simulink model "xxxx"  (R2025a)
settings: Solver=ode23t  StartTime=0.0  StopTime=10.0  RelTol=1e-3  AbsTol=1e-3  EnableMultiTasking=on
values from neighbouring files (symbols this model uses):
  FemurHeight = 0.25    [xxxx_ini.m]
  FemurRadius = 0.05    [xxxx_ini.m]
  FootDepth = 0.25    [xxxx_ini.m]
  FootHeight = 0.05    [xxxx_ini.m]
  FootWidth = 0.1    [xxxx_ini.m]
  PelvisHorizontalPositionInit = FemurHeight * sin(HipRadInit)                               + TibiaHeight * sin(HipRadInit + KneeRadInit)    [xxxx_ini.m]
  PelvisRadius = 0.15    [xxxx_ini.m]
  PelvisVerticalPositionInit = FemurHeight * cos(HipRadInit)                             + TibiaHeight * cos(HipRadInit + KneeRadInit)                             + FootHeight                             + FootRadius    [xxxx_ini.m]
  TibiaHeight = 0.25    [xxxx_ini.m]
undefined symbols (not defined in the file or in its folder): PelvisWidth, X, Y, Z
libraries: sm_lib x55, nesl_utility x35, rllib x1, simulink x1
(part 2 of 2)

== system xxxx/Body/HipJoint_L1 ==
  PS-Simulink Converter : nesl_utility/PS-Simulink Converter  PhysicalDomain=network_engine_domain  SubClassName=ps_output  LeftPortType=input  RightPortType=output  PseudoPeriodic=off  Frequencies=[]  VectorFormat=inherit  Unit=inherit  AffineConversion=off
  PS-Simulink Converter1 : nesl_utility/PS-Simulink Converter  PhysicalDomain=network_engine_domain  SubClassName=ps_output  LeftPortType=input  RightPortType=output  PseudoPeriodic=off  Frequencies=[]  VectorFormat=inherit  Unit=inherit  AffineConversion=off
  PS-Simulink Converter2 : nesl_utility/PS-Simulink Converter  PhysicalDomain=network_engine_domain  SubClassName=ps_output  LeftPortType=input  RightPortType=output  PseudoPeriodic=off  Frequencies=[]  VectorFormat=inherit  Unit=inherit  AffineConversion=off
  Revolute Joint : sm_lib/Joints/Revolute Joint  JointMode=Normal  CompositeWrenchDir=FollowerOnBase  CompositeWrenchFrame=BaseFrame  SenseConstraintForce=off  SenseConstraintTorque=off  SenseTotalForce=off  SenseTotalTorque=off  PositionTargetSpecify=on  PositionTargetPriority=High  PositionTargetValue=HipDegInit  PositionTargetValueUnits=deg  VelocityTargetSpecify=off  VelocityTargetPriority=High  VelocityTargetValue=0  VelocityTargetValueUnits=deg/s  EquilibriumPosition=0  EquilibriumPositionUnits=deg  SpringStiffness=0  SpringStiffnessUnits=N*m/deg  DampingCoefficient=0  DampingCoefficientUnits=N*m/(deg/s)  LowerLimitSpecify=on  LowerLimitBound=0  LowerLimitBoundUnits=deg  LowerLimitStiffness=1e4  LowerLimitStiffnessUnits=N*m/deg  LowerLimitDamping=10  LowerLimitDampingUnits=N*m/(deg/s)  LowerLimitTransitionRegionWidth=0.1  LowerLimitTransitionRegionWidthUnits=deg  UpperLimitSpecify=on  UpperLimitBound=90  UpperLimitBoundUnits=deg  UpperLimitStiffness=1e4  UpperLimitStiffnessUnits=N*m/deg  UpperLimitDamping=10  UpperLimitDampingUnits=N*m/(deg/s)  UpperLimitTransitionRegionWidth=0.1  UpperLimitTransitionRegionWidthUnits=deg  TorqueActuationMode=InputTorque  MotionActuationMode=ComputedMotion  SensePosition=on  SenseVelocity=on  SenseAcceleration=on  SenseTorqueForce=off  SenseLowerLimitTorqueForce=off  SenseUpperLimitTorqueForce=off
  Rigid Transform : sm_lib/Frames and Transforms/Rigid Transform  RotationMethod=StandardAxis  FollAlignAxisA=+X  BaseAlignAxisA=+Y  FollAlignAxisB=+Y  BaseAlignAxisB=+Z  RotationStandardAxis=-Y  RotationAngle=90  RotationAngleUnits=deg  RotationArbitraryAxis=[0 0 1]  RotationSequenceAxes=FollowerAxes  RotationSequence=XYX  RotationSequenceAngles=[0 0 0]  RotationSequenceAnglesUnits=deg  RotationMatrix=[1 0 0;0 1 0;0 0 1]  Quaternion=[1 0 0 0]  TranslationMethod=StandardAxis  TranslationCartesianOffset=[-(PelvisRadius + FemurRadius) 0 0 ]  TranslationCartesianOffsetUnits=m  TranslationStandardAxis=+X  TranslationStandardOffset=PelvisRadius + FemurRadius  TranslationStandardOffsetUnits=m  TranslationROffset=0  TranslationROffsetUnits=m  TranslationThetaOffset=0  TranslationThetaOffsetUnits=deg  TranslationZOffset=0  TranslationZOffsetUnits=m
  Rigid Transform2 : sm_lib/Frames and Transforms/Rigid Transform  RotationMethod=StandardAxis  FollAlignAxisA=+X  BaseAlignAxisA=+Y  FollAlignAxisB=+Y  BaseAlignAxisB=+Z  RotationStandardAxis=+Y  RotationAngle=90  RotationAngleUnits=deg  RotationArbitraryAxis=[0 0 1]  RotationSequenceAxes=FollowerAxes  RotationSequence=XYX  RotationSequenceAngles=[0 0 0]  RotationSequenceAnglesUnits=deg  RotationMatrix=[1 0 0;0 1 0;0 0 1]  Quaternion=[1 0 0 0]  TranslationMethod=StandardAxis  TranslationCartesianOffset=[0 0 0]  TranslationCartesianOffsetUnits=m  TranslationStandardAxis=-X  TranslationStandardOffset=FemurHeight/2  TranslationStandardOffsetUnits=m  TranslationROffset=0  TranslationROffsetUnits=m  TranslationThetaOffset=0  TranslationThetaOffsetUnits=deg  TranslationZOffset=0  TranslationZOffsetUnits=m
  Simulink-PS Converter : nesl_utility/Simulink-PS Converter  PhysicalDomain=network_engine_domain  SubClassName=ps_input  LeftPortType=input  RightPortType=output  PseudoPeriodic=off  Frequencies=[]  NoiseDistribution=none  NoiseParameters=[]  Unit=1  AffineConversion=off  FilteringAndDerivatives=provide  SimscapeFilterOrder=1  InputFilterTimeConstant=0.001  UdotUserProvided=0
  R : PMIOPort  Side=Left
  H : PMIOPort  Port=2  Side=Right
  tag scope: HipAcc_R=global, HipPos_R=global, HipVel_R=global
  wires:
  [HipTorque_R] -> Simulink-PS Converter/1
  PS-Simulink Converter2/1 -> [HipAcc_R]
  PS-Simulink Converter1/1 -> [HipVel_R]
  PS-Simulink Converter/1 -> [HipPos_R]
  connections:
  Simulink-PS Converter/RConn1 -- Revolute Joint/LConn2
  PS-Simulink Converter2/LConn1 -- Revolute Joint/RConn4
  PS-Simulink Converter1/LConn1 -- Revolute Joint/RConn3
  PS-Simulink Converter/LConn1 -- Revolute Joint/RConn2
  Revolute Joint/RConn1 -- Rigid Transform2/LConn1
  Rigid Transform/RConn1 -- Revolute Joint/LConn1
  Rigid Transform2/RConn1 -- H/RConn1
  R/RConn1 -- Rigid Transform/LConn1

== system xxxx/Body/KneeJoint_L ==
  PS-Simulink Converter : nesl_utility/PS-Simulink Converter  PhysicalDomain=network_engine_domain  SubClassName=ps_output  LeftPortType=input  RightPortType=output  PseudoPeriodic=off  Frequencies=[]  VectorFormat=inherit  Unit=inherit  AffineConversion=off
  PS-Simulink Converter1 : nesl_utility/PS-Simulink Converter  PhysicalDomain=network_engine_domain  SubClassName=ps_output  LeftPortType=input  RightPortType=output  PseudoPeriodic=off  Frequencies=[]  VectorFormat=inherit  Unit=inherit  AffineConversion=off
  PS-Simulink Converter2 : nesl_utility/PS-Simulink Converter  PhysicalDomain=network_engine_domain  SubClassName=ps_output  LeftPortType=input  RightPortType=output  PseudoPeriodic=off  Frequencies=[]  VectorFormat=inherit  Unit=inherit  AffineConversion=off
  Revolute Joint : sm_lib/Joints/Revolute Joint  JointMode=Normal  CompositeWrenchDir=FollowerOnBase  CompositeWrenchFrame=BaseFrame  SenseConstraintForce=off  SenseConstraintTorque=off  SenseTotalForce=off  SenseTotalTorque=off  PositionTargetSpecify=on  PositionTargetPriority=High  PositionTargetValue=KneeDegInit  PositionTargetValueUnits=deg  VelocityTargetSpecify=off  VelocityTargetPriority=High  VelocityTargetValue=0  VelocityTargetValueUnits=deg/s  EquilibriumPosition=0  EquilibriumPositionUnits=deg  SpringStiffness=0  SpringStiffnessUnits=N*m/deg  DampingCoefficient=0  DampingCoefficientUnits=N*m/(deg/s)  LowerLimitSpecify=on  LowerLimitBound=0  LowerLimitBoundUnits=deg  LowerLimitStiffness=1e4  LowerLimitStiffnessUnits=N*m/deg  LowerLimitDamping=10  LowerLimitDampingUnits=N*m/(deg/s)  LowerLimitTransitionRegionWidth=0.1  LowerLimitTransitionRegionWidthUnits=deg  UpperLimitSpecify=on  UpperLimitBound=90  UpperLimitBoundUnits=deg  UpperLimitStiffness=1e4  UpperLimitStiffnessUnits=N*m/deg  UpperLimitDamping=10  UpperLimitDampingUnits=N*m/(deg/s)  UpperLimitTransitionRegionWidth=0.1  UpperLimitTransitionRegionWidthUnits=deg  TorqueActuationMode=InputTorque  MotionActuationMode=ComputedMotion  SensePosition=on  SenseVelocity=on  SenseAcceleration=on  SenseTorqueForce=off  SenseLowerLimitTorqueForce=off  SenseUpperLimitTorqueForce=off
  Rigid Transform : sm_lib/Frames and Transforms/Rigid Transform  RotationMethod=StandardAxis  FollAlignAxisA=+X  BaseAlignAxisA=+Y  FollAlignAxisB=+Y  BaseAlignAxisB=+Z  RotationStandardAxis=-Y  RotationAngle=90  RotationAngleUnits=deg  RotationArbitraryAxis=[0 0 1]  RotationSequenceAxes=FollowerAxes  RotationSequence=XYX  RotationSequenceAngles=[0 0 0]  RotationSequenceAnglesUnits=deg  RotationMatrix=[1 0 0;0 1 0;0 0 1]  Quaternion=[1 0 0 0]  TranslationMethod=StandardAxis  TranslationCartesianOffset=[0 0 0]  TranslationCartesianOffsetUnits=m  TranslationStandardAxis=-Z  TranslationStandardOffset=FemurHeight/2  TranslationStandardOffsetUnits=m  TranslationROffset=0  TranslationROffsetUnits=m  TranslationThetaOffset=0  TranslationThetaOffsetUnits=deg  TranslationZOffset=0  TranslationZOffsetUnits=m
  Rigid Transform1 : sm_lib/Frames and Transforms/Rigid Transform  RotationMethod=StandardAxis  FollAlignAxisA=+X  BaseAlignAxisA=+Y  FollAlignAxisB=+Y  BaseAlignAxisB=+Z  RotationStandardAxis=+Y  RotationAngle=90  RotationAngleUnits=deg  RotationArbitraryAxis=[0 0 1]  RotationSequenceAxes=FollowerAxes  RotationSequence=XYX  RotationSequenceAngles=[0 0 0]  RotationSequenceAnglesUnits=deg  RotationMatrix=[1 0 0;0 1 0;0 0 1]  Quaternion=[1 0 0 0]  TranslationMethod=StandardAxis  TranslationCartesianOffset=[0 0 0]  TranslationCartesianOffsetUnits=m  TranslationStandardAxis=-X  TranslationStandardOffset=TibiaHeight/2  TranslationStandardOffsetUnits=m  TranslationROffset=0  TranslationROffsetUnits=m  TranslationThetaOffset=0  TranslationThetaOffsetUnits=deg  TranslationZOffset=0  TranslationZOffsetUnits=m
  Simulink-PS Converter : nesl_utility/Simulink-PS Converter  PhysicalDomain=network_engine_domain  SubClassName=ps_input  LeftPortType=input  RightPortType=output  PseudoPeriodic=off  Frequencies=[]  NoiseDistribution=none  NoiseParameters=[]  Unit=1  AffineConversion=off  FilteringAndDerivatives=provide  SimscapeFilterOrder=1  InputFilterTimeConstant=0.001  UdotUserProvided=0
  R : PMIOPort  Side=Left
  H : PMIOPort  Port=2  Side=Right
  tag scope: KneeAcc_L=global, KneePos_L=global, KneeVel_L=global
  wires:
  PS-Simulink Converter1/1 -> [KneeVel_L]
  PS-Simulink Converter2/1 -> [KneeAcc_L]
  PS-Simulink Converter/1 -> [KneePos_L]
  [KneeTorque_L] -> Simulink-PS Converter/1
  connections:
  PS-Simulink Converter/LConn1 -- Revolute Joint/RConn2
  PS-Simulink Converter1/LConn1 -- Revolute Joint/RConn3
  PS-Simulink Converter2/LConn1 -- Revolute Joint/RConn4
  Simulink-PS Converter/RConn1 -- Revolute Joint/LConn2
  R/RConn1 -- Rigid Transform/LConn1
  H/RConn1 -- Rigid Transform1/RConn1
  Rigid Transform/RConn1 -- Revolute Joint/LConn1
  Rigid Transform1/LConn1 -- Revolute Joint/RConn1

== system xxxx/Body/KneeJoint_L1 ==
  PS-Simulink Converter : nesl_utility/PS-Simulink Converter  PhysicalDomain=network_engine_domain  SubClassName=ps_output  LeftPortType=input  RightPortType=output  PseudoPeriodic=off  Frequencies=[]  VectorFormat=inherit  Unit=inherit  AffineConversion=off
  PS-Simulink Converter1 : nesl_utility/PS-Simulink Converter  PhysicalDomain=network_engine_domain  SubClassName=ps_output  LeftPortType=input  RightPortType=output  PseudoPeriodic=off  Frequencies=[]  VectorFormat=inherit  Unit=inherit  AffineConversion=off
  PS-Simulink Converter2 : nesl_utility/PS-Simulink Converter  PhysicalDomain=network_engine_domain  SubClassName=ps_output  LeftPortType=input  RightPortType=output  PseudoPeriodic=off  Frequencies=[]  VectorFormat=inherit  Unit=inherit  AffineConversion=off
  Revolute Joint : sm_lib/Joints/Revolute Joint  JointMode=Normal  CompositeWrenchDir=FollowerOnBase  CompositeWrenchFrame=BaseFrame  SenseConstraintForce=off  SenseConstraintTorque=off  SenseTotalForce=off  SenseTotalTorque=off  PositionTargetSpecify=on  PositionTargetPriority=High  PositionTargetValue=KneeDegInit  PositionTargetValueUnits=deg  VelocityTargetSpecify=off  VelocityTargetPriority=High  VelocityTargetValue=0  VelocityTargetValueUnits=deg/s  EquilibriumPosition=0  EquilibriumPositionUnits=deg  SpringStiffness=0  SpringStiffnessUnits=N*m/deg  DampingCoefficient=0  DampingCoefficientUnits=N*m/(deg/s)  LowerLimitSpecify=on  LowerLimitBound=0  LowerLimitBoundUnits=deg  LowerLimitStiffness=1e4  LowerLimitStiffnessUnits=N*m/deg  LowerLimitDamping=10  LowerLimitDampingUnits=N*m/(deg/s)  LowerLimitTransitionRegionWidth=0.1  LowerLimitTransitionRegionWidthUnits=deg  UpperLimitSpecify=on  UpperLimitBound=90  UpperLimitBoundUnits=deg  UpperLimitStiffness=1e4  UpperLimitStiffnessUnits=N*m/deg  UpperLimitDamping=10  UpperLimitDampingUnits=N*m/(deg/s)  UpperLimitTransitionRegionWidth=0.1  UpperLimitTransitionRegionWidthUnits=deg  TorqueActuationMode=InputTorque  MotionActuationMode=ComputedMotion  SensePosition=on  SenseVelocity=on  SenseAcceleration=on  SenseTorqueForce=off  SenseLowerLimitTorqueForce=off  SenseUpperLimitTorqueForce=off
  Rigid Transform : sm_lib/Frames and Transforms/Rigid Transform  RotationMethod=StandardAxis  FollAlignAxisA=+X  BaseAlignAxisA=+Y  FollAlignAxisB=+Y  BaseAlignAxisB=+Z  RotationStandardAxis=-Y  RotationAngle=90  RotationAngleUnits=deg  RotationArbitraryAxis=[0 0 1]  RotationSequenceAxes=FollowerAxes  RotationSequence=XYX  RotationSequenceAngles=[0 0 0]  RotationSequenceAnglesUnits=deg  RotationMatrix=[1 0 0;0 1 0;0 0 1]  Quaternion=[1 0 0 0]  TranslationMethod=StandardAxis  TranslationCartesianOffset=[0 0 0]  TranslationCartesianOffsetUnits=m  TranslationStandardAxis=-Z  TranslationStandardOffset=FemurHeight/2  TranslationStandardOffsetUnits=m  TranslationROffset=0  TranslationROffsetUnits=m  TranslationThetaOffset=0  TranslationThetaOffsetUnits=deg  TranslationZOffset=0  TranslationZOffsetUnits=m
  Rigid Transform1 : sm_lib/Frames and Transforms/Rigid Transform  RotationMethod=StandardAxis  FollAlignAxisA=+X  BaseAlignAxisA=+Y  FollAlignAxisB=+Y  BaseAlignAxisB=+Z  RotationStandardAxis=+Y  RotationAngle=90  RotationAngleUnits=deg  RotationArbitraryAxis=[0 0 1]  RotationSequenceAxes=FollowerAxes  RotationSequence=XYX  RotationSequenceAngles=[0 0 0]  RotationSequenceAnglesUnits=deg  RotationMatrix=[1 0 0;0 1 0;0 0 1]  Quaternion=[1 0 0 0]  TranslationMethod=StandardAxis  TranslationCartesianOffset=[0 0 0]  TranslationCartesianOffsetUnits=m  TranslationStandardAxis=-X  TranslationStandardOffset=TibiaHeight/2  TranslationStandardOffsetUnits=m  TranslationROffset=0  TranslationROffsetUnits=m  TranslationThetaOffset=0  TranslationThetaOffsetUnits=deg  TranslationZOffset=0  TranslationZOffsetUnits=m
  Simulink-PS Converter : nesl_utility/Simulink-PS Converter  PhysicalDomain=network_engine_domain  SubClassName=ps_input  LeftPortType=input  RightPortType=output  PseudoPeriodic=off  Frequencies=[]  NoiseDistribution=none  NoiseParameters=[]  Unit=1  AffineConversion=off  FilteringAndDerivatives=provide  SimscapeFilterOrder=1  InputFilterTimeConstant=0.001  UdotUserProvided=0
  R : PMIOPort  Side=Left
  H : PMIOPort  Port=2  Side=Right
  tag scope: KneeAcc_R=global, KneePos_R=global, KneeVel_R=global
  wires:
  [KneeTorque_R] -> Simulink-PS Converter/1
  PS-Simulink Converter/1 -> [KneePos_R]
  PS-Simulink Converter2/1 -> [KneeAcc_R]
  PS-Simulink Converter1/1 -> [KneeVel_R]
  connections:
  Rigid Transform1/LConn1 -- Revolute Joint/RConn1
  Rigid Transform/RConn1 -- Revolute Joint/LConn1
  H/RConn1 -- Rigid Transform1/RConn1
  R/RConn1 -- Rigid Transform/LConn1
  Simulink-PS Converter/RConn1 -- Revolute Joint/LConn2
  PS-Simulink Converter2/LConn1 -- Revolute Joint/RConn4
  PS-Simulink Converter1/LConn1 -- Revolute Joint/RConn3
  PS-Simulink Converter/LConn1 -- Revolute Joint/RConn2

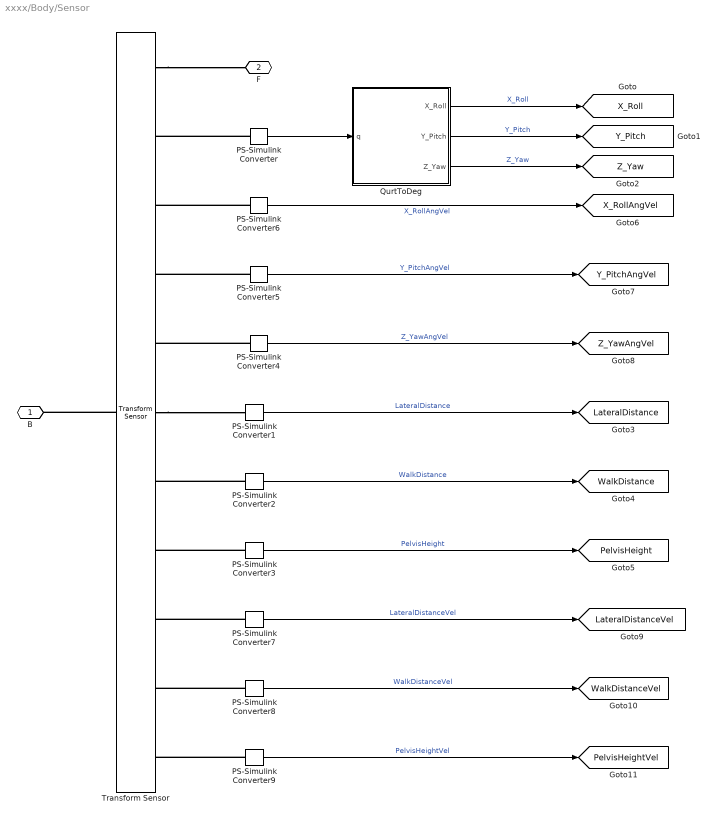
== system xxxx/Body/Sensor ==
  PS-Simulink Converter{,1..9} (10 alike) : nesl_utility/PS-Simulink Converter  PhysicalDomain=network_engine_domain  SubClassName=ps_output  LeftPortType=input  RightPortType=output  PseudoPeriodic=off  Frequencies=[]  VectorFormat=inherit  Unit=inherit  AffineConversion=off
  QurtToDeg : Subsystem
  Transform Sensor : sm_lib/Frames and Transforms/Transform Sensor  MeasurementFrame=World  RotationSequence=ZYX  SenseAngle=off  SenseAxis=off  SenseQ=on  SenseR=off  SenseRotationSequence=off  SenseOmegaX=on  SenseOmegaY=on  SenseOmegaZ=on  SenseOmega=off  SenseQDot=off  SenseRDot=off  SenseRotationSequenceDot=off  SenseAlphaX=off  SenseAlphaY=off  SenseAlphaZ=off  SenseAlpha=off  SenseQDDot=off  SenseRDDot=off  SenseX=on  SenseY=on  SenseZ=on  SenseXYZ=off  SenseRad=off  SenseAzim=off  SenseDist=off  SenseInc=off  SenseXDot=on  SenseYDot=on  SenseZDot=on  SenseXYZDot=off  SenseRadDot=off  SenseAzimDot=off  SenseDistDot=off  SenseIncDot=off  SenseXDDot=off  SenseYDDot=off  SenseZDDot=off  SenseXYZDDot=off  SenseRadDDot=off  SenseAzimDDot=off  SenseDistDDot=off  SenseIncDDot=off
  B : PMIOPort  Side=Left
  F : PMIOPort  Port=2  Side=Right
  tag scope: LateralDistance=global, LateralDistanceVel=global, PelvisHeight=global, PelvisHeightVel=global, WalkDistance=global, WalkDistanceVel=global, X_Roll=global, X_RollAngVel=global, Y_Pitch=global, Y_PitchAngVel=global, Z_Yaw=global, Z_YawAngVel=global
  wires:
  PS-Simulink Converter/1 -> QurtToDeg/1(q)
  PS-Simulink Converter1/1 -> [LateralDistance]  "LateralDistance"
  PS-Simulink Converter2/1 -> [WalkDistance]  "WalkDistance"
  PS-Simulink Converter3/1 -> [PelvisHeight]  "PelvisHeight"
  QurtToDeg/1(X_Roll) -> [X_Roll]  "X_Roll"
  QurtToDeg/2(Y_Pitch) -> [Y_Pitch]  "Y_Pitch"
  QurtToDeg/3(Z_Yaw) -> [Z_Yaw]  "Z_Yaw"
  PS-Simulink Converter5/1 -> [Y_PitchAngVel]  "Y_PitchAngVel"
  PS-Simulink Converter6/1 -> [X_RollAngVel]  "X_RollAngVel"
  PS-Simulink Converter4/1 -> [Z_YawAngVel]  "Z_YawAngVel"
  PS-Simulink Converter9/1 -> [PelvisHeightVel]  "PelvisHeightVel"
  PS-Simulink Converter8/1 -> [WalkDistanceVel]  "WalkDistanceVel"
  PS-Simulink Converter7/1 -> [LateralDistanceVel]  "LateralDistanceVel"
  connections:
  PS-Simulink Converter2/LConn1 -- Transform Sensor/RConn7
  Transform Sensor/RConn1 -- F/RConn1
  Transform Sensor/LConn1 -- B/RConn1
  PS-Simulink Converter3/LConn1 -- Transform Sensor/RConn8
  PS-Simulink Converter/LConn1 -- Transform Sensor/RConn2
  Transform Sensor/RConn6 -- PS-Simulink Converter1/LConn1
  PS-Simulink Converter4/LConn1 -- Transform Sensor/RConn5
  PS-Simulink Converter5/LConn1 -- Transform Sensor/RConn4
  PS-Simulink Converter6/LConn1 -- Transform Sensor/RConn3
  PS-Simulink Converter7/LConn1 -- Transform Sensor/RConn9
  PS-Simulink Converter8/LConn1 -- Transform Sensor/RConn10
  PS-Simulink Converter9/LConn1 -- Transform Sensor/RConn11

== system xxxx/Body/Tibia_L ==
  Cylindrical Solid : sm_lib/Body Elements/Cylindrical Solid  CylinderRadius=TibiaRadius  CylinderRadiusUnits=m  CylinderLength=TibiaHeight  CylinderLengthUnits=m  ExportEntireGeometry=off  InertiaType=CalculateFromGeometry  BasedOnType=Density  Density=Dencity  DensityUnits=kg/m^3  Mass=1  MassUnits=kg  CenterOfMass=[0 0 0]  CenterOfMassUnits=m  MomentsOfInertia=[1 1 1]  MomentsOfInertiaUnits=kg*m^2  ProductsOfInertia=[0 0 0]  ProductsOfInertiaUnits=kg*m^2  GraphicType=FromGeometry  MarkerShape=Sphere  MarkerSize=10  GraphicVisPropType=SimpleVisualProperties  GraphicDiffuseColor=[0.5 0.5 0.5]  GraphicOpacity=1  GraphicSpecularColor=[0.5 0.5 0.5 1.0]  GraphicAmbientColor=[0.15 0.15 0.15 1.0]  GraphicEmissiveColor=[0.0 0.0 0.0 1.0]  GraphicShininess=75  DoExposeReferenceFrame=on  SerializedFrames=<Frames/>
  R : PMIOPort  Side=Left
  H : PMIOPort  Port=2  Side=Right
  connections:
  Cylindrical Solid/RConn1 -- H/RConn1 -- R/RConn1

== system xxxx/Body/Tibia_L1 ==
  Cylindrical Solid : sm_lib/Body Elements/Cylindrical Solid  CylinderRadius=TibiaRadius  CylinderRadiusUnits=m  CylinderLength=TibiaHeight  CylinderLengthUnits=m  ExportEntireGeometry=off  InertiaType=CalculateFromGeometry  BasedOnType=Density  Density=Dencity  DensityUnits=kg/m^3  Mass=1  MassUnits=kg  CenterOfMass=[0 0 0]  CenterOfMassUnits=m  MomentsOfInertia=[1 1 1]  MomentsOfInertiaUnits=kg*m^2  ProductsOfInertia=[0 0 0]  ProductsOfInertiaUnits=kg*m^2  GraphicType=FromGeometry  MarkerShape=Sphere  MarkerSize=10  GraphicVisPropType=SimpleVisualProperties  GraphicDiffuseColor=[0.5 0.5 0.5]  GraphicOpacity=1  GraphicSpecularColor=[0.5 0.5 0.5 1.0]  GraphicAmbientColor=[0.15 0.15 0.15 1.0]  GraphicEmissiveColor=[0.0 0.0 0.0 1.0]  GraphicShininess=75  DoExposeReferenceFrame=on  SerializedFrames=<Frames/>
  R : PMIOPort  Side=Left
  H : PMIOPort  Port=2  Side=Right
  connections:
  H/RConn1 -- R/RConn1 -- Cylindrical Solid/RConn1

== system xxxx/Body/WorldFrame ==
  Infinite Plane : sm_lib/Curves and Surfaces/Infinite Plane  GraphicType=Rectangle  GraphicPlaneWidth=1  GraphicPlaneWidthUnits=m  GraphicPlaneHeight=1  GraphicPlaneHeightUnits=m  GraphicVisPropType=SimpleVisualProperties  GraphicDiffuseColor=[0.5 0.5 0.5]  GraphicOpacity=1  GraphicSpecularColor=[0.5 0.5 0.5 1.0]  GraphicAmbientColor=[0.15 0.15 0.15 1.0]  GraphicEmissiveColor=[0.0 0.0 0.0 1.0]  GraphicShininess=75
  Mechanism Configuration : sm_lib/Utilities/Mechanism Configuration  UniformGravity=Constant  GravityVector=[0 0 -9.80665]  GravityVectorUnits=m/s^2  LinearizationDelta=0.001  JointModeTransitionNonlinearIterations=2
  Solver Configuration : nesl_utility/Solver Configuration  PhysicalDomain=network_engine_domain  SubClassName=solver  LeftPortType=input  RightPortType=generic  Tones=[]  Harmonics=[]  SimulateNoise=off  Profile=off  UseLocalSampling=off  EnableSwitchedLinearOptims=on  FrequencyDomain=off  UseCCode=off  RelTol=0.001  AbsTol=1e-06  MinStep=1e-09  ToWorkspace=off  RevertToSquareIcSolve=off  NumHomotopyIterations=100  PhasorMode=off  PhasorModeNumHarmonics=1  ConsistencySolver=NEWTON_XTOL_AFTER_FTOL  IndexReductionMethod=DerivativeReplacement  DoDC=off  ResidualTolerance=1e-09  ConsistencyTolSource=GLOBAL  ConsistencyAbsTol=0.001  ConsistencyRelTol=0.001  ConsistencyTolFactor=0.001  UseLocalSolver=off  LocalSolverChoice=NE_BACKWARD_EULER_ADVANCER  ResolveIndetEquations=on  FunctionEvalNumThread=1  LocalSolverSampleTime=0.001  DoFixedCost=off  MaxNonlinIter=3  MaxModeIter=2  ComputeImpulses=off  ImpulseIterations=2  LinearAlgebra=Sparse  LinearAlgebraNumThread=0  EquationFormulation=NE_TIME_EF  DelaysMemoryBudget=1024  AutomaticFiltering=on  FilteringTimeConstant=0.001  PartitionStorageMethod=AS_NEEDED  PartitionMemoryBudget=1024  PartitionMethod=FAST  MultibodyUseLocalSolver=off  MultibodyLocalSolverChoice=ODE1  MultibodyLocalSolverSampleTime=0.001
  World Frame : sm_lib/Frames and Transforms/World Frame
  R : PMIOPort  Side=Right
  G : PMIOPort  Port=2  Side=Right
  connections:
  World Frame/RConn1 -- Solver Configuration/RConn1 -- Infinite Plane/LConn1 -- R/RConn1 -- Mechanism Configuration/RConn1
  G/RConn1 -- Infinite Plane/RConn1

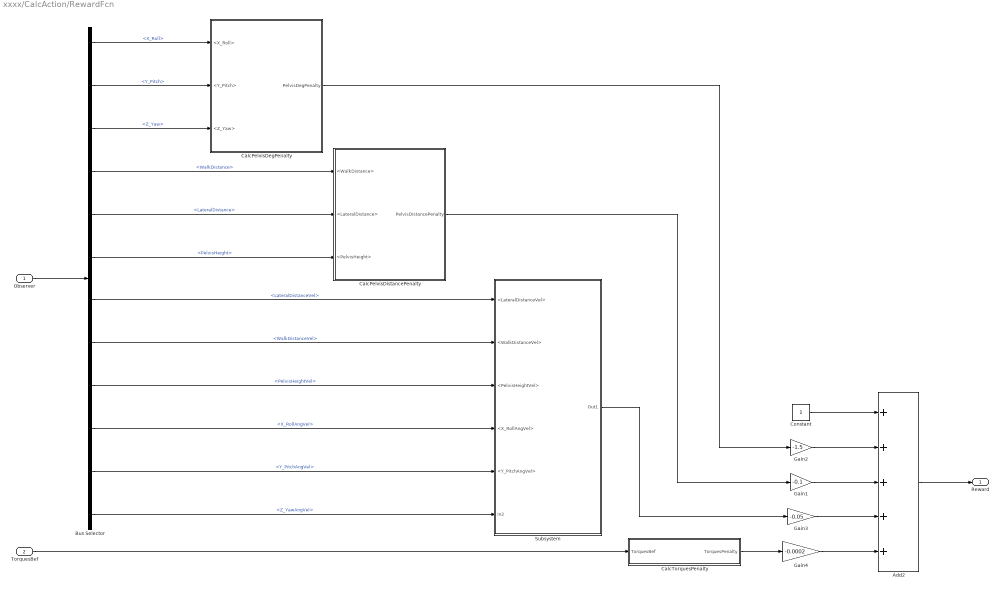
== system xxxx/CalcAction/RewardFcn ==
  Observer : Inport
  TorquesBef : Inport  Port=2
  Add2 : Sum  Inputs=+++++
  Bus Selector : BusSelector  OutputSignals=X_Roll,Y_Pitch,Z_Yaw,WalkDistance,LateralDistance,PelvisHeight,LateralDistanceVel,WalkDistanceVel,PelvisHeightVel,X_RollAngVel,Y_PitchAngVel,Z_YawAngVel
  CalcPelvisDegPenalty : Subsystem
  CalcPelvisDistancePenalty : Subsystem
  CalcTorquesPenalty : Subsystem
  Constant : Constant
  Gain1 : Gain  Gain=-0.1
  Gain2 : Gain  Gain=-1.5
  Gain3 : Gain  Gain=-0.05
  Gain4 : Gain  Gain=-0.0002
  Subsystem : Subsystem
  Reward : Outport
  wires:
  Observer/1 -> Bus Selector/1
  Bus Selector/1 -> CalcPelvisDegPenalty/1(<X_Roll>)  "<X_Roll>"
  Bus Selector/2 -> CalcPelvisDegPenalty/2(<Y_Pitch>)  "<Y_Pitch>"
  Bus Selector/3 -> CalcPelvisDegPenalty/3(<Z_Yaw>)  "<Z_Yaw>"
  CalcPelvisDegPenalty/1(PelvisDegPenalty) -> Gain2/1
  Bus Selector/4 -> CalcPelvisDistancePenalty/1(<WalkDistance>)  "<WalkDistance>"
  Bus Selector/5 -> CalcPelvisDistancePenalty/2(<LateralDistance>)  "<LateralDistance>"
  Bus Selector/6 -> CalcPelvisDistancePenalty/3(<PelvisHeight>)  "<PelvisHeight>"
  CalcPelvisDistancePenalty/1(PelvisDistancePenalty) -> Gain1/1
  Bus Selector/7 -> Subsystem/1(<LateralDistanceVel>)  "<LateralDistanceVel>"
  Bus Selector/8 -> Subsystem/2(<WalkDistanceVel>)  "<WalkDistanceVel>"
  Bus Selector/11 -> Subsystem/5(<Y_PitchAngVel>)  "<Y_PitchAngVel>"
  Bus Selector/10 -> Subsystem/4(<X_RollAngVel>)  "<X_RollAngVel>"
  Subsystem/1(Out1) -> Gain3/1
  Add2/1 -> Reward/1
  Bus Selector/9 -> Subsystem/3(<PelvisHeightVel>)  "<PelvisHeightVel>"
  Bus Selector/12 -> Subsystem/6(In2)  "<Z_YawAngVel>"
  TorquesBef/1 -> CalcTorquesPenalty/1(TorquesBef)
  CalcTorquesPenalty/1(TorquesPenalty) -> Gain4/1
  Gain3/1 -> Add2/4
  Gain1/1 -> Add2/3
  Constant/1 -> Add2/1
  Gain2/1 -> Add2/2
  Gain4/1 -> Add2/5

== system xxxx/CalcAction/isDoneFcn ==
  Observer : Inport
  Bus Selector : BusSelector  OutputSignals=PelvisHeight
  Compare To Constant : simulink/Logic and Bit Operations/Compare To Constant  relop=<=  const=0  OutDataTypeStr=boolean
  isDone : Outport
  wires:
  Bus Selector/1 -> Compare To Constant/1  "<PelvisHeight>"
  Observer/1 -> Bus Selector/1
  Compare To Constant/1 -> isDone/1

== system xxxx/Body/Sensor/QurtToDeg ==
  q : Inport
  Demux : Demux
  Gain1 : Gain  Gain=180/pi
  Gain2 : Gain  Gain=180/pi
  Gain3 : Gain  Gain=180/pi
  Subsystem : Subsystem
  Subsystem1 : Subsystem
  Subsystem2 : Subsystem
  X_Roll : Outport
  Y_Pitch : Outport  Port=2
  Z_Yaw : Outport  Port=3
  wires:
  Demux/1 -> Subsystem2/1(w), Subsystem1/1(w), Subsystem/1(w)  "w"
  Demux/2 -> Subsystem2/2(x), Subsystem1/2(x), Subsystem/2(x)  "x"
  Demux/3 -> Subsystem2/3(y), Subsystem1/3(y), Subsystem/3(y)  "y"
  Demux/4 -> Subsystem2/4(z), Subsystem1/4(z), Subsystem/4(z)  "z"
  Subsystem/1(Roll) -> Gain1/1
  Subsystem1/1(Pitch) -> Gain2/1
  Subsystem2/1(Yaw) -> Gain3/1
  q/1 -> Demux/1
  Gain1/1 -> X_Roll/1  "Roll"
  Gain2/1 -> Y_Pitch/1  "Pitch"
  Gain3/1 -> Z_Yaw/1  "Yaw"

== system xxxx/CalcAction/RewardFcn/CalcPelvisDegPenalty ==
  <X_Roll> : Inport
  <Y_Pitch> : Inport  Port=2
  <Z_Yaw> : Inport  Port=3
  Add : Sum  Inputs=+++
  Gain : Gain  Gain=1/180
  Gain3 : Gain  Gain=1/180
  Gain4 : Gain  Gain=1/180
  Square : Math  Operator=square
  Square1 : Math  Operator=square
  Square2 : Math  Operator=square
  PelvisDegPenalty : Outport
  wires:
  <X_Roll>/1 -> Gain/1
  Square/1 -> Add/1
  Gain/1 -> Square/1
  Square2/1 -> Add/3
  Square1/1 -> Add/2
  Gain3/1 -> Square1/1
  Gain4/1 -> Square2/1
  <Y_Pitch>/1 -> Gain3/1
  <Z_Yaw>/1 -> Gain4/1
  Add/1 -> PelvisDegPenalty/1

== system xxxx/CalcAction/RewardFcn/CalcPelvisDistancePenalty ==
  <WalkDistance> : Inport
  <LateralDistance> : Inport  Port=2
  <PelvisHeight> : Inport  Port=3
  Add1 : Sum  Inputs=+++
  Square3 : Math  Operator=square
  Square4 : Math  Operator=square
  Square5 : Math  Operator=square
  Subsystem : Subsystem
  Subsystem1 : Subsystem
  PelvisDistancePenalty : Outport
  wires:
  Square3/1 -> Add1/1
  <PelvisHeight>/1 -> Subsystem1/1(<PelvisHeight>)
  Add1/1 -> PelvisDistancePenalty/1
  Square5/1 -> Add1/3
  Subsystem/1(Out1) -> Square3/1
  Square4/1 -> Add1/2
  Subsystem1/1(Out1) -> Square5/1
  <LateralDistance>/1 -> Square4/1
  <WalkDistance>/1 -> Subsystem/1(<WalkDistance>)

== system xxxx/CalcAction/RewardFcn/CalcTorquesPenalty ==
  TorquesBef : Inport
  Square : Math  Operator=square
  Sum of Elements : Sum  Inputs=+
  TorquesPenalty : Outport
  wires:
  Sum of Elements/1 -> TorquesPenalty/1
  Square/1 -> Sum of Elements/1
  TorquesBef/1 -> Square/1

== system xxxx/CalcAction/RewardFcn/Subsystem ==
  <LateralDistanceVel> : Inport
  <WalkDistanceVel> : Inport  Port=2
  <PelvisHeightVel> : Inport  Port=3
  <X_RollAngVel> : Inport  Port=4
  <Y_PitchAngVel> : Inport  Port=5
  In2 : Inport  Port=6
  Add : Sum  Inputs=++++++
  Square{,1..4} (5 alike) : Math  Operator=square
  Out1 : Outport
  wires:
  Square1/1 -> Add/2
  <WalkDistanceVel>/1 -> Square1/1
  Add/1 -> Out1/1
  <X_RollAngVel>/1 -> Square3/1
  Square/1 -> Add/1
  <LateralDistanceVel>/1 -> Square/1
  <Y_PitchAngVel>/1 -> Square2/1
  <PelvisHeightVel>/1 -> Square4/1
  Square4/1 -> Add/3
  Square2/1 -> Add/5
  Square3/1 -> Add/4

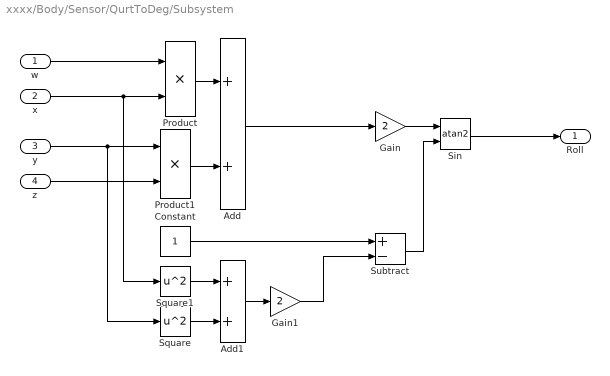
== system xxxx/Body/Sensor/QurtToDeg/Subsystem ==
  w : Inport
  x : Inport  Port=2
  y : Inport  Port=3
  z : Inport  Port=4
  Add : Sum
  Add1 : Sum
  Constant : Constant
  Gain : Gain  Gain=2
  Gain1 : Gain  Gain=2
  Product : Product
  Product1 : Product
  Sin : Trigonometry  Operator=atan2
  Square : Math  Operator=square
  Square1 : Math  Operator=square
  Subtract : Sum  Inputs=+-
  Roll : Outport
  wires:
  Subtract/1 -> Sin/2
  Constant/1 -> Subtract/1
  z/1 -> Product1/2
  y/1 -> Square/1, Product1/1
  Add/1 -> Gain/1
  Square/1 -> Add1/2
  Add1/1 -> Gain1/1
  Square1/1 -> Add1/1
  x/1 -> Square1/1, Product/2
  Gain/1 -> Sin/1
  Product/1 -> Add/1
  Product1/1 -> Add/2
  w/1 -> Product/1
  Sin/1 -> Roll/1
  Gain1/1 -> Subtract/2

== system xxxx/Body/Sensor/QurtToDeg/Subsystem1 ==
  w : Inport
  x : Inport  Port=2
  y : Inport  Port=3
  z : Inport  Port=4
  Add : Sum
  Gain : Gain  Gain=2
  Product : Product
  Product1 : Product
  Saturation : Saturate  UpperLimit=1  LowerLimit=-1
  Sin : Trigonometry  Operator=asin
  Pitch : Outport
  wires:
  w/1 -> Product/1
  Product1/1 -> Add/2
  Product/1 -> Add/1
  Gain/1 -> Saturation/1
  Add/1 -> Gain/1
  z/1 -> Product1/2
  y/1 -> Product/2
  x/1 -> Product1/1
  Sin/1 -> Pitch/1
  Saturation/1 -> Sin/1

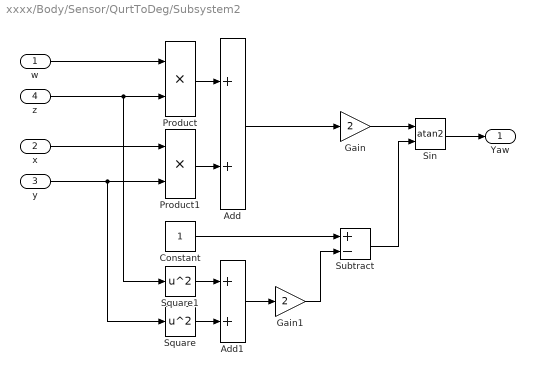
== system xxxx/Body/Sensor/QurtToDeg/Subsystem2 ==
  w : Inport
  x : Inport  Port=2
  y : Inport  Port=3
  z : Inport  Port=4
  Add : Sum
  Add1 : Sum
  Constant : Constant
  Gain : Gain  Gain=2
  Gain1 : Gain  Gain=2
  Product : Product
  Product1 : Product
  Sin : Trigonometry  Operator=atan2
  Square : Math  Operator=square
  Square1 : Math  Operator=square
  Subtract : Sum  Inputs=+-
  Yaw : Outport
  wires:
  Subtract/1 -> Sin/2
  Constant/1 -> Subtract/1
  Add/1 -> Gain/1
  Square/1 -> Add1/2
  Add1/1 -> Gain1/1
  Square1/1 -> Add1/1
  z/1 -> Square1/1, Product/2
  Gain/1 -> Sin/1
  Product/1 -> Add/1
  Product1/1 -> Add/2
  w/1 -> Product/1
  Sin/1 -> Yaw/1
  x/1 -> Product1/1
  y/1 -> Product1/2, Square/1
  Gain1/1 -> Subtract/2

== system xxxx/CalcAction/RewardFcn/CalcPelvisDistancePenalty/Subsystem ==
  <WalkDistance> : Inport
  Constant1 : Constant  Value=PelvisHorizontalPositionInit
  Subtract1 : Sum  Inputs=+-
  Out1 : Outport
  wires:
  Constant1/1 -> Subtract1/2
  <WalkDistance>/1 -> Subtract1/1
  Subtract1/1 -> Out1/1

== system xxxx/CalcAction/RewardFcn/CalcPelvisDistancePenalty/Subsystem1 ==
  <PelvisHeight> : Inport
  Constant : Constant  Value=PelvisVerticalPositionInit
  Subtract : Sum  Inputs=+-
  Out1 : Outport
  wires:
  Constant/1 -> Subtract/2
  Subtract/1 -> Out1/1
  <PelvisHeight>/1 -> Subtract/1
